simulink model "regulator_LQR_discrete_Ueq"  (Simulink 10.0)
settings: Solver=ode45  StartTime=0.0  StopTime=tsim  RelTol=1e-3  EnableMultiTasking=on
values from neighbouring files (symbols this model uses):
  C_states = eye(2)    [es3.m]
  D_states = [0 0]'    [es3.m]
  Klqr1 = dlqr(A,B,Q,R)    [es3.m]
  sat_max = inf    [es3.m]
  sat_min = -inf    [es3.m]
  Ts = 0.1    [es3.m]
  Ubar = inv(dcgain(Gz))*Ybar    [es3.m]
  x0 = [5 20]    [es3.m]
  xref = Xbar    [es3.m]
undefined symbols (not defined in the file or in its folder): A, B, C
settings Model: Creator=Administrator  LastModifiedBy=Chiara
settings DataIOCC: LimitDataPoints=on  SignalLoggingSaveFormat=ModelDataLogs
settings OptimizationCC: ExpressionDepthLimit=2147483647  InitFltsAndDblsToZero=on
settings DebuggingCC: SolverPrmCheckMsg=warning  FcnCallInpInsideContextMsg=warning  StateNameClashWarn=warning
settings GRTTargetCC: GeneratePreprocessorConditionals=Disable all
settings ConfigComp: CovExternalEMLEnable=off  CovSFcnEnable=off

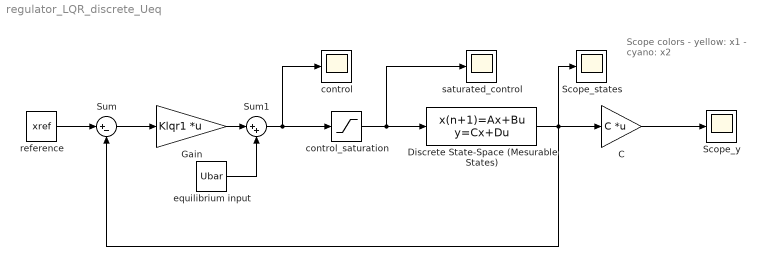
== system regulator_LQR_discrete_Ueq ==
  note: Scope colors
      | - yellow: x1
      | - cyano: x2
  C : Gain  Gain=C  Multiplication=Matrix(K*u)
  Discrete State-Space (Mesurable States) : DiscreteStateSpace  A=A  B=B  C=C_states  D=D_states  InitialCondition=x0  SampleTime=Ts
  Gain : Gain  Gain=Klqr1  Multiplication=Matrix(K*u)
  Scope_states : Scope
  Scope_y : Scope
  Sum : Sum  Inputs=|+-
  Sum1 : Sum  Inputs=|++
  control : Scope
  control_saturation : Saturate  UpperLimit=sat_max  LowerLimit=sat_min
  equilibrium input : Constant  Value=Ubar
  reference : Constant  Value=xref
  saturated_control : Scope
  wires:
  control_saturation/1 -> Discrete State-Space (Mesurable States)/1, saturated_control/1
  Sum/1 -> Gain/1
  Discrete State-Space (Mesurable States)/1 -> C/1, Scope_states/1, Sum/2
  C/1 -> Scope_y/1
  Gain/1 -> Sum1/1
  Sum1/1 -> control/1, control_saturation/1
  equilibrium input/1 -> Sum1/2
  reference/1 -> Sum/1
